simulink model "dvbs2hdlTransmitterCore"  (R2024b)
settings: Solver=FixedStepDiscrete  StartTime=0.0  StopTime=0  RelTol=1e-3
libraries: hdlsllib x105, simulink x41, dspsigops x7, commseqgen3 x5, whdlutilities x5, commhdlcrc x2, dsphdlfiltering2 x1, whdlmod x1
(part 1 of 5)
settings Model: DataDictionary=dvbs2hdlReceiverData.sldd  DataTypeOverride=Off  Creator=The MathWorks, Inc.  LastModifiedBy=daniel
settings SolverCC: MaxZcPerStep=1
settings OptimizationCC: BlockReduction=off  ConditionallyExecuteInputs=off  DefaultParameterBehavior=Inlined  InheritOutputTypeSmallerThanSingle=on  ReuseModelBlockBuffer=off
settings DebuggingCC: AlgebraicLoopMsg=error  SingleTaskRateTransMsg=error  SubsystemReferenceDiagnosticForUnitTest=warning
settings HardwareCC: ProdBitPerPointer=32  ProdBitPerSizeT=32  ProdBitPerPtrDiffT=32  ProdLargestAtomicFloat=None  ProdIntDivRoundTo=Undefined  ProdEndianess=Unspecified  ProdWordSize=32  ProdHWDeviceType=ASIC/FPGA->ASIC/FPGA  TargetBitPerLong=64  TargetBitPerPointer=64  TargetBitPerSizeT=64  TargetBitPerPtrDiffT=64  TargetLongLongMode=on  TargetIntDivRoundTo=Zero  TargetEndianess=LittleEndian  TargetWordSize=64  TargetHWDeviceType=Custom Processor->MATLAB Host Computer  ProdEqTarget=off
settings ModelReferenceCC: EnableRefExpFcnMdlSchedulingChecks=on
settings RTWCC: GPUComputeCapability=3.5  DLArmComputeVersion=19.05

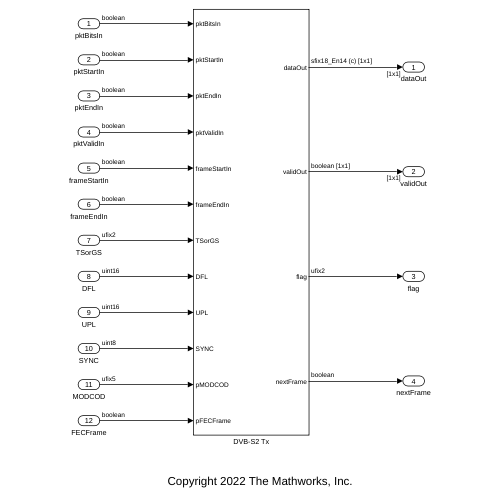
[thumbnail: Simulink's stored preview of the top-level diagram]
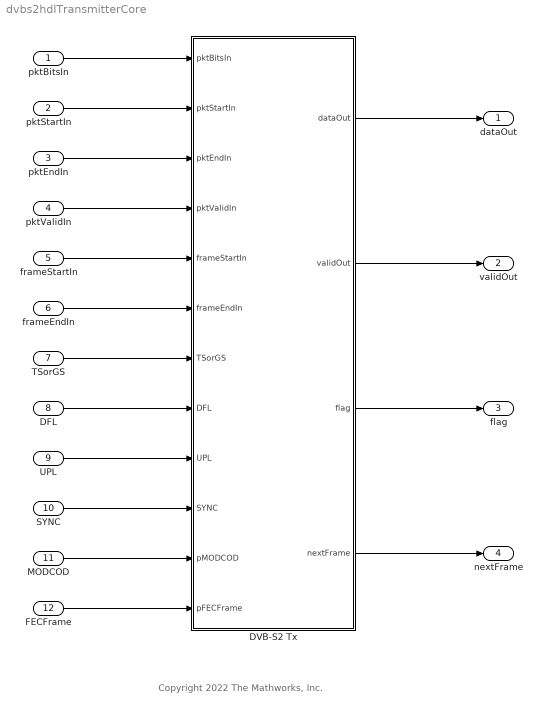
== system dvbs2hdlTransmitterCore ==
  note: Copyright 2022 The Mathworks, Inc.
  pktBitsIn : Inport  OutDataTypeStr=boolean  PortDimensions=1
  pktStartIn : Inport  Port=2  OutDataTypeStr=boolean  PortDimensions=1
  pktEndIn : Inport  Port=3  OutDataTypeStr=boolean  PortDimensions=1
  pktValidIn : Inport  Port=4  OutDataTypeStr=boolean  PortDimensions=1
  frameStartIn : Inport  Port=5  OutDataTypeStr=boolean  PortDimensions=1
  frameEndIn : Inport  Port=6  OutDataTypeStr=boolean  PortDimensions=1
  TSorGS : Inport  Port=7  OutDataTypeStr=fixdt(0,2,0)  PortDimensions=1
  DFL : Inport  Port=8  OutDataTypeStr=uint16  PortDimensions=1
  UPL : Inport  Port=9  OutDataTypeStr=uint16  PortDimensions=1
  SYNC : Inport  Port=10  OutDataTypeStr=uint8  PortDimensions=1
  MODCOD : Inport  Port=11  OutDataTypeStr=fixdt(0,5,0)  PortDimensions=1
  FECFrame : Inport  Port=12  OutDataTypeStr=boolean  PortDimensions=1
  DVB-S2 Tx : Subsystem  mask{Rsym=5e6}
      mask prompts: Rsym "Symbol Rate:"
      mask init:
      | config = dvbs2hdlTxParameters();
  dataOut : Outport
  validOut : Outport  Port=2
  flag : Outport  Port=3
  nextFrame : Outport  Port=4
  wires:
  pktBitsIn/1 -> DVB-S2 Tx/1(pktBitsIn)
  pktStartIn/1 -> DVB-S2 Tx/2(pktStartIn)
  pktEndIn/1 -> DVB-S2 Tx/3(pktEndIn)
  pktValidIn/1 -> DVB-S2 Tx/4(pktValidIn)
  frameStartIn/1 -> DVB-S2 Tx/5(frameStartIn)
  frameEndIn/1 -> DVB-S2 Tx/6(frameEndIn)
  TSorGS/1 -> DVB-S2 Tx/7(TSorGS)
  DFL/1 -> DVB-S2 Tx/8(DFL)
  UPL/1 -> DVB-S2 Tx/9(UPL)
  SYNC/1 -> DVB-S2 Tx/10(SYNC)
  MODCOD/1 -> DVB-S2 Tx/11(pMODCOD)
  FECFrame/1 -> DVB-S2 Tx/12(pFECFrame)
  DVB-S2 Tx/4(nextFrame) -> nextFrame/1
  DVB-S2 Tx/2(validOut) -> validOut/1
  DVB-S2 Tx/1(dataOut) -> dataOut/1
  DVB-S2 Tx/3(flag) -> flag/1

== system dvbs2hdlTransmitterCore/DVB-S2 Tx ==
  pktBitsIn : Inport  SampleTime=1/(Rsym*8)
  pktStartIn : Inport  Port=2
  pktEndIn : Inport  Port=3
  pktValidIn : Inport  Port=4
  frameStartIn : Inport  Port=5
  frameEndIn : Inport  Port=6
  TSorGS : Inport  Port=7
  DFL : Inport  Port=8
  UPL : Inport  Port=9
  SYNC : Inport  Port=10
  pMODCOD : Inport  Port=11
  pFECFrame : Inport  Port=12
  BB Frame Generator : Subsystem
  Bit Concat : hdlsllib/Logic and Bit Operations/Bit Concat  numInputs=2
  Delay : Delay  DelayLength=1
  FEC Encoder : Subsystem
  Interleaver : Subsystem
  Logical Operator : Logic  Operator=NOT  AllPortsSameDT=off  OutDataTypeStr=boolean
  Logical Operator1 : Logic  AllPortsSameDT=off  OutDataTypeStr=boolean
  MODCOD Source Coder : Subsystem
  No HDL : Subsystem
  PL Frame Generator : Subsystem
  RRC Transmit Filter : Subsystem
  Symbol Modulator : Subsystem
  Unit Delay Enabled Resettable Synchronous : hdlsllib/Discrete/Unit Delay Enabled Resettable Synchronous  InitialCondition=0.0  SampleTime=-1
  dataOut : Outport
  validOut : Outport  Port=2
  flag : Outport  Port=3
  nextFrame : Outport  Port=4
  wires:
  BB Frame Generator/4(validOut) -> MODCOD Source Coder/4(validIn)
  Delay/1 -> Logical Operator/1
  Logical Operator/1 -> Logical Operator1/2
  Logical Operator1/1 -> Unit Delay Enabled Resettable Synchronous/2, Unit Delay Enabled Resettable Synchronous/1
  PL Frame Generator/4(PLHeaderEnd) -> Bit Concat/2, No HDL/2(enb)
  PL Frame Generator/3(dummyHeaderEnd) -> Bit Concat/1, No HDL/1(Enable)
  Interleaver/8(MODCOD) -> Symbol Modulator/8(MODCOD)
  Interleaver/7(modIdx) -> Symbol Modulator/7(modIdx)
  Interleaver/6(codIdx) -> Symbol Modulator/6(codIdx)
  Interleaver/5(FECFrame) -> Symbol Modulator/5(FECFrame)
  Interleaver/4(validOut) -> Symbol Modulator/4(validIn)
  Interleaver/3(endOut) -> Symbol Modulator/3(endIn)
  Interleaver/2(startOut) -> Symbol Modulator/2(startIn)
  Interleaver/1(dataOut) -> Symbol Modulator/1(dataIn)
  FEC Encoder/7(MODCOD) -> Interleaver/7(MODCODIn)
  FEC Encoder/5(codOut) -> Interleaver/5(codIdxIn)
  FEC Encoder/2(validOut) -> Interleaver/2(validIn)
  FEC Encoder/1(dataOut) -> Interleaver/1(dataIn)
  PL Frame Generator/2(validOut) -> RRC Transmit Filter/2(validIn)
  PL Frame Generator/1(dataOut) -> RRC Transmit Filter/1(dataIn)
  Symbol Modulator/8(MODCODOut) -> PL Frame Generator/8(modcod)
  Symbol Modulator/7(FECFrameOut) -> PL Frame Generator/7(fecframeIn)
  Symbol Modulator/6(codIdxOut) -> PL Frame Generator/6(codIdxIn)
  Symbol Modulator/5(modIdxOut) -> PL Frame Generator/5(modIdxIn)
  Symbol Modulator/4(validOut) -> PL Frame Generator/4(validIn)
  Symbol Modulator/3(endOut) -> PL Frame Generator/3(endIn)
  Symbol Modulator/2(startOut) -> PL Frame Generator/2(startIn)
  Symbol Modulator/1(dataOut) -> PL Frame Generator/1(dataIn)
  RRC Transmit Filter/2(validOut) -> validOut/1
  RRC Transmit Filter/1(dataOut) -> dataOut/1
  pFECFrame/1 -> BB Frame Generator/12(pFECFrame)
  Interleaver/9(ready) -> Delay/1, Logical Operator1/1
  frameEndIn/1 -> BB Frame Generator/6(frameEndIn)
  TSorGS/1 -> BB Frame Generator/7(TSorGS)
  pktBitsIn/1 -> BB Frame Generator/1(pktBitsIn)
  pktEndIn/1 -> BB Frame Generator/3(pktEndIn)
  DFL/1 -> BB Frame Generator/8(DFL)
  FEC Encoder/3(startOut) -> Interleaver/3(paramValid)
  MODCOD Source Coder/4(validOut) -> FEC Encoder/4(validIn)
  pktValidIn/1 -> BB Frame Generator/4(pktValidIn)
  MODCOD Source Coder/1(dataOut) -> FEC Encoder/1(dataIn)
  MODCOD Source Coder/3(endOut) -> FEC Encoder/3(endIn)
  MODCOD Source Coder/8(MODCOD) -> FEC Encoder/8(MODCODIn)
  BB Frame Generator/6(FECFrame) -> MODCOD Source Coder/6(FECFrameIn)
  BB Frame Generator/1(dataOut) -> MODCOD Source Coder/1(dataIn)
  pMODCOD/1 -> BB Frame Generator/11(pMODCOD)
  MODCOD Source Coder/2(startOut) -> FEC Encoder/2(startIn)
  MODCOD Source Coder/6(codeRateIdx) -> FEC Encoder/6(codeRateIdxIn)
  SYNC/1 -> BB Frame Generator/10(SYNC)
  UPL/1 -> BB Frame Generator/9(UPL)
  BB Frame Generator/2(startOut) -> MODCOD Source Coder/2(startIn)
  pktStartIn/1 -> BB Frame Generator/2(pktStartIn)
  BB Frame Generator/5(MODCOD) -> MODCOD Source Coder/5(MODCODIn)
  MODCOD Source Coder/5(modIdx) -> FEC Encoder/5(modIdxIn)
  MODCOD Source Coder/7(FECFrame) -> FEC Encoder/7(FECFrameIn)
  frameStartIn/1 -> Unit Delay Enabled Resettable Synchronous/3, BB Frame Generator/5(frameStartIn)
  FEC Encoder/4(modOut) -> Interleaver/4(modIdxIn)
  BB Frame Generator/3(endOut) -> MODCOD Source Coder/3(endIn)
  FEC Encoder/6(fecOut) -> Interleaver/6(fecframeIn)
  Unit Delay Enabled Resettable Synchronous/1 -> nextFrame/1
  Bit Concat/1 -> flag/1

== system dvbs2hdlTransmitterCore/DVB-S2 Tx/BB Frame Generator ==
  pktBitsIn : Inport
  pktStartIn : Inport  Port=2
  pktEndIn : Inport  Port=3
  pktValidIn : Inport  Port=4
  frameStartIn : Inport  Port=5
  frameEndIn : Inport  Port=6
  TSorGS : Inport  Port=7
  DFL : Inport  Port=8
  UPL : Inport  Port=9
  SYNC : Inport  Port=10
  pMODCOD : Inport  Port=11
  pFECFrame : Inport  Port=12
  BB Header and Data CRC Generator : Subsystem
  BB Scrambler : Subsystem
  Data Store FIFO : Subsystem
  Delay{,1..5} (6 alike) : Delay  DelayLength=1
  Multiplexer : Subsystem
  Unit Delay Enabled Synchronous{,1..5} (6 alike) : hdlsllib/Discrete/Unit Delay Enabled Synchronous  InitialCondition=0.0  SampleTime=-1
  dataOut : Outport
  startOut : Outport  Port=2
  endOut : Outport  Port=3
  validOut : Outport  Port=4
  MODCOD : Outport  Port=5
  FECFrame : Outport  Port=6
  wires:
  BB Scrambler/6(FECFrameOut) -> FECFrame/1
  Multiplexer/6(FECFrameOut) -> BB Scrambler/6(FECFrame)
  Data Store FIFO/8(FECFrameOut) -> Multiplexer/8(FECFrame)
  BB Header and Data CRC Generator/9(FECFrameOut) -> Data Store FIFO/9(FECFrame)
  Unit Delay Enabled Synchronous5/1 -> BB Header and Data CRC Generator/12(FECFrame)
  pFECFrame/1 -> Unit Delay Enabled Synchronous5/1
  BB Scrambler/5(MODCODOut) -> MODCOD/1
  Multiplexer/5(MODCODOut) -> BB Scrambler/5(MODCOD)
  Data Store FIFO/7(MODCODOut) -> Multiplexer/7(MODCOD)
  BB Header and Data CRC Generator/8(MODCODOut) -> Data Store FIFO/8(MODCOD)
  pMODCOD/1 -> Unit Delay Enabled Synchronous4/1
  Unit Delay Enabled Synchronous4/1 -> BB Header and Data CRC Generator/11(MODCOD)
  BB Header and Data CRC Generator/7(validOut) -> Data Store FIFO/7(validOut)
  BB Header and Data CRC Generator/6(endOut) -> Data Store FIFO/6(endOut)
  BB Header and Data CRC Generator/5(startOut) -> Data Store FIFO/5(startOut)
  BB Header and Data CRC Generator/4(bitsOut) -> Data Store FIFO/4(bitsOut)
  Data Store FIFO/6(headerValid) -> Multiplexer/6(headerValid)
  Data Store FIFO/5(headerStart) -> Multiplexer/5(headerStart)
  Data Store FIFO/4(headerBits) -> Multiplexer/4(headerBits)
  Data Store FIFO/3(dataEnd) -> Multiplexer/3(dataEnd)
  Data Store FIFO/2(dataValid) -> Multiplexer/2(dataValid)
  Data Store FIFO/1(dataBits) -> Multiplexer/1(dataBits)
  BB Header and Data CRC Generator/3(DFLOut) -> Data Store FIFO/3(DFLOut)
  BB Header and Data CRC Generator/2(pktValid) -> Data Store FIFO/2(pktValid)
  BB Header and Data CRC Generator/1(pktBits) -> Data Store FIFO/1(pktBits)
  Unit Delay Enabled Synchronous3/1 -> BB Header and Data CRC Generator/10(SYNC)
  Unit Delay Enabled Synchronous2/1 -> BB Header and Data CRC Generator/9(UPL)
  Unit Delay Enabled Synchronous/1 -> BB Header and Data CRC Generator/8(DFL)
  Unit Delay Enabled Synchronous1/1 -> BB Header and Data CRC Generator/7(TSorGS)
  Delay2/1 -> BB Header and Data CRC Generator/6(frameStart)
  Delay/1 -> BB Header and Data CRC Generator/5(frameEnd)
  Delay1/1 -> BB Header and Data CRC Generator/4(validIn)
  Delay3/1 -> BB Header and Data CRC Generator/3(endIn)
  Delay4/1 -> BB Header and Data CRC Generator/2(startIn)
  Delay5/1 -> BB Header and Data CRC Generator/1(dataIn)
  BB Scrambler/4(validOut) -> validOut/1
  BB Scrambler/3(endOut) -> endOut/1
  BB Scrambler/2(startOut) -> startOut/1
  BB Scrambler/1(bitsOut) -> dataOut/1
  Multiplexer/1(dataOut) -> BB Scrambler/1(bitsIn)
  Multiplexer/3(endOut) -> BB Scrambler/3(endIn)
  Multiplexer/2(startOut) -> BB Scrambler/2(startIn)
  Multiplexer/4(validOut) -> BB Scrambler/4(validIn)
  frameStartIn/1 -> Delay2/1, Unit Delay Enabled Synchronous1/2, Unit Delay Enabled Synchronous/2, Unit Delay Enabled Synchronous2/2, Unit Delay Enabled Synchronous3/2, Unit Delay Enabled Synchronous4/2, Unit Delay Enabled Synchronous5/2
  pktBitsIn/1 -> Delay5/1
  pktStartIn/1 -> Delay4/1
  pktEndIn/1 -> Delay3/1
  pktValidIn/1 -> Delay1/1
  frameEndIn/1 -> Delay/1
  DFL/1 -> Unit Delay Enabled Synchronous/1
  UPL/1 -> Unit Delay Enabled Synchronous2/1
  SYNC/1 -> Unit Delay Enabled Synchronous3/1
  TSorGS/1 -> Unit Delay Enabled Synchronous1/1

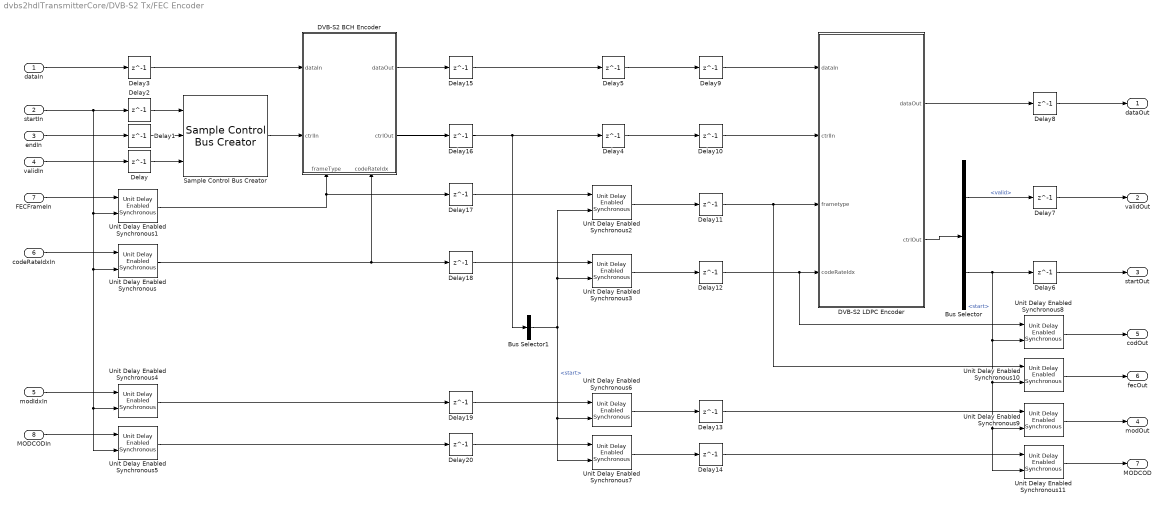
== system dvbs2hdlTransmitterCore/DVB-S2 Tx/FEC Encoder ==
  dataIn : Inport
  startIn : Inport  Port=2
  endIn : Inport  Port=3
  validIn : Inport  Port=4
  modIdxIn : Inport  Port=5
  codeRateIdxIn : Inport  Port=6
  FECFrameIn : Inport  Port=7
  MODCODIn : Inport  Port=8
  Bus Selector : BusSelector  OutputSignals=valid,start
  Bus Selector1 : BusSelector  OutputSignals=start
  DVB-S2 BCH Encoder : Subsystem
      settings: PortSchema="{\"entries\":[{\"content\":{\"sides\":[{\"content\":{\"connectorIds\":[\"In1\",\"In2\"]},\"type\":\"ConnectorPlacement.EquallySpacedRectSide\",\"uuid\":\"13af3286-4637-4d72-a307-8c85e9ac2c6a\"},{\"content\":{\"connectorIds\":[\"Out1\",\"Out2\"],\"side\":\"RIGHT\"},\"type\":\"ConnectorPlacement.EquallySpacedRectSide\",\"uuid\":\"54f73aa5-b2da-4ba3-a1a2-5182494cfccf\"},{\"content\":{\"connectorIds\":[],\"side\":\"TOP\"},\"type\":\"ConnectorPlacement.EquallySpacedRectSide\",\"uuid\":\"2ea82380-bfbe-4164-83be-b799e77a8d24\"},{\"content\":{\"connectorIds\":[\"In3\",\"In4\"],\"side\":\"BOTTOM\"},\"type\":\"ConnectorPlacement.EquallySpacedRectSide\",\"uuid\":\"b02c2a1c-1695-4c1d-92ad-7323b1632720\"}]},\"type\":\"ConnectorPlacement.EquallySpacedConnector\",\"uuid\":\"56402870-0df7-4074-88cd-682c42d8a6b3\"}],\"packageUris\":[\"http://schema.mathworks.com/mf0/Connector/R2020b\"],\"version\":\"1.0\"}"
  DVB-S2 LDPC Encoder : Subsystem
      mask init:
      | config = dvbs2hdlTxParameters();
      | columnSum = config.LDPCcolumnSum;  %#ok<NASGU> 
      | ramLUT    = config.LDPCramLUT;     %#ok<NASGU> 
      | shiftLUT  = config.LDPCshiftLUT;   %#ok<NASGU>
  Delay{,1..20} (21 alike) : Delay  DelayLength=1
  Sample Control Bus Creator : whdlutilities/Sample Control Bus Creator
  Unit Delay Enabled Synchronous{,1..11} (12 alike) : hdlsllib/Discrete/Unit Delay Enabled Synchronous  InitialCondition=0.0  SampleTime=-1
  dataOut : Outport
  validOut : Outport  Port=2
  startOut : Outport  Port=3
  modOut : Outport  Port=4
  codOut : Outport  Port=5
  fecOut : Outport  Port=6
  MODCOD : Outport  Port=7
  wires:
  Delay20/1 -> Unit Delay Enabled Synchronous7/1
  Delay19/1 -> Unit Delay Enabled Synchronous6/1
  Delay18/1 -> Unit Delay Enabled Synchronous3/1
  Delay17/1 -> Unit Delay Enabled Synchronous2/1
  Delay16/1 -> Delay4/1, Bus Selector1/1
  Delay15/1 -> Delay5/1
  Delay14/1 -> Unit Delay Enabled Synchronous11/1
  Delay13/1 -> Unit Delay Enabled Synchronous9/1
  Delay12/1 -> DVB-S2 LDPC Encoder/4(codeRateIdx), Unit Delay Enabled Synchronous8/1
  Delay11/1 -> DVB-S2 LDPC Encoder/3(frametype), Unit Delay Enabled Synchronous10/1
  Delay10/1 -> DVB-S2 LDPC Encoder/2(ctrlIn)
  Delay9/1 -> DVB-S2 LDPC Encoder/1(dataIn)
  validIn/1 -> Delay/1
  endIn/1 -> Delay1/1
  startIn/1 -> Delay2/1, Unit Delay Enabled Synchronous1/2, Unit Delay Enabled Synchronous/2, Unit Delay Enabled Synchronous4/2, Unit Delay Enabled Synchronous5/2
  Delay3/1 -> DVB-S2 BCH Encoder/1(dataIn)
  Unit Delay Enabled Synchronous1/1 -> Delay17/1, DVB-S2 BCH Encoder/3(frameType)
  Unit Delay Enabled Synchronous/1 -> DVB-S2 BCH Encoder/4(codeRateIdx), Delay18/1
  Sample Control Bus Creator/1 -> DVB-S2 BCH Encoder/2(ctrlIn)
  DVB-S2 BCH Encoder/2(ctrlOut) -> Delay16/1
  DVB-S2 BCH Encoder/1(dataOut) -> Delay15/1
  Unit Delay Enabled Synchronous3/1 -> Delay12/1
  Delay8/1 -> dataOut/1
  Delay7/1 -> validOut/1
  Delay6/1 -> startOut/1
  Delay5/1 -> Delay9/1
  Delay4/1 -> Delay10/1
  Delay2/1 -> Sample Control Bus Creator/1
  Delay1/1 -> Sample Control Bus Creator/2
  Delay/1 -> Sample Control Bus Creator/3
  Unit Delay Enabled Synchronous7/1 -> Delay14/1
  Unit Delay Enabled Synchronous6/1 -> Delay13/1
  Unit Delay Enabled Synchronous11/1 -> MODCOD/1
  Unit Delay Enabled Synchronous10/1 -> fecOut/1
  Unit Delay Enabled Synchronous9/1 -> modOut/1
  Unit Delay Enabled Synchronous8/1 -> codOut/1
  Unit Delay Enabled Synchronous5/1 -> Delay20/1
  Unit Delay Enabled Synchronous4/1 -> Delay19/1
  MODCODIn/1 -> Unit Delay Enabled Synchronous5/1
  Unit Delay Enabled Synchronous2/1 -> Delay11/1
  Bus Selector1/1 -> Unit Delay Enabled Synchronous6/2, Unit Delay Enabled Synchronous7/2, Unit Delay Enabled Synchronous3/2, Unit Delay Enabled Synchronous2/2  "<start>"
  dataIn/1 -> Delay3/1
  codeRateIdxIn/1 -> Unit Delay Enabled Synchronous/1
  FECFrameIn/1 -> Unit Delay Enabled Synchronous1/1
  modIdxIn/1 -> Unit Delay Enabled Synchronous4/1
  Bus Selector/2 -> Delay6/1, Unit Delay Enabled Synchronous8/2, Unit Delay Enabled Synchronous10/2, Unit Delay Enabled Synchronous9/2, Unit Delay Enabled Synchronous11/2  "<start>"
  Bus Selector/1 -> Delay7/1  "<valid>"
  DVB-S2 LDPC Encoder/2(ctrlOut) -> Bus Selector/1
  DVB-S2 LDPC Encoder/1(dataOut) -> Delay8/1

== system dvbs2hdlTransmitterCore/DVB-S2 Tx/Interleaver ==
  dataIn : Inport
  validIn : Inport  Port=2
  paramValid : Inport  Port=3
  modIdxIn : Inport  Port=4
  codIdxIn : Inport  Port=5
  fecframeIn : Inport  Port=6
  MODCODIn : Inport  Port=7
  DVB-S2 HDL Interleaver : Subsystem  mask{mode=Interleaver 8x, Tsamp=1/(Rsym*8)}
      mask prompts: mode "Mode :"; Tsamp "Sample Time"
      mask init:
      | switch mode
      |     case 1
      |         isInterleave = true;
      |     case 2
      |         isInterleave = false;
      |     otherwise
      |         error(['Invalid mode of ' mode]);
      | end
      | clear mode;
      | 
      | ConfigRx.RAMCapacity = 64800*2;
      | ConfigRx.ShortFrameLen = 16200;
      | ConfigRx.NormalFrameLen = 64800;
      mask TypeOptions mode: Interleaver 8x | Deinterleaver
      mask Display: disp(['DVB-S2' newline 'HDL ' newline get_param(gcb,'mode')]);
  Delay{1,3..5,17..20} (8 alike) : Delay  DelayLength=8
  Delay{2,6..13} (9 alike) : Delay  DelayLength=1
  Unit Delay Enabled Synchronous : hdlsllib/Discrete/Unit Delay Enabled Synchronous  InitialCondition=0.0  SampleTime=-1
  dataOut : Outport
  startOut : Outport  Port=2
  endOut : Outport  Port=3
  validOut : Outport  Port=4
  FECFrame : Outport  Port=5
  codIdx : Outport  Port=6
  modIdx : Outport  Port=7
  MODCOD : Outport  Port=8
  ready : Outport  Port=9
  wires:
  Delay1/1 -> endOut/1
  fecframeIn/1 -> DVB-S2 HDL Interleaver/6(fecframeIn)
  modIdxIn/1 -> DVB-S2 HDL Interleaver/4(modIdxIn)
  codIdxIn/1 -> DVB-S2 HDL Interleaver/5(codIdxIn)
  Delay4/1 -> validOut/1
  DVB-S2 HDL Interleaver/8(ready) -> ready/1
  MODCODIn/1 -> Unit Delay Enabled Synchronous/1
  Delay17/1 -> FECFrame/1
  Delay5/1 -> startOut/1
  Delay10/1 -> DVB-S2 HDL Interleaver/2(validIn)
  Delay19/1 -> dataOut/1
  Delay12/1 -> Delay18/1
  dataIn/1 -> Delay9/1
  Delay20/1 -> modIdx/1
  DVB-S2 HDL Interleaver/1(rd_dout) -> Delay2/1
  Delay11/1 -> Delay17/1
  validIn/1 -> Delay10/1
  Delay9/1 -> DVB-S2 HDL Interleaver/1(dataIn)
  Delay8/1 -> Delay4/1
  Delay2/1 -> Delay19/1
  Unit Delay Enabled Synchronous/1 -> Delay3/1
  DVB-S2 HDL Interleaver/2(rd_startOut) -> Delay6/1, Unit Delay Enabled Synchronous/2
  DVB-S2 HDL Interleaver/6(codIdx) -> Delay12/1
  DVB-S2 HDL Interleaver/3(rd_endOut) -> Delay7/1
  Delay3/1 -> MODCOD/1
  Delay6/1 -> Delay5/1
  Delay18/1 -> codIdx/1
  DVB-S2 HDL Interleaver/7(modIdx) -> Delay13/1
  Delay7/1 -> Delay1/1
  paramValid/1 -> DVB-S2 HDL Interleaver/3(paramValid)
  DVB-S2 HDL Interleaver/4(rd_validOut) -> Delay8/1
  DVB-S2 HDL Interleaver/5(fecframe) -> Delay11/1
  Delay13/1 -> Delay20/1

== system dvbs2hdlTransmitterCore/DVB-S2 Tx/MODCOD Source Coder ==
  dataIn : Inport
  startIn : Inport  Port=2
  endIn : Inport  Port=3
  validIn : Inport  Port=4
  MODCODIn : Inport  Port=5
  FECFrameIn : Inport  Port=6
  Data Type Conversion : DataTypeConversion  OutDataTypeStr=fixdt(0,4,0)  SaturateOnIntegerOverflow=off  RndMeth=Floor
  Data Type Conversion1 : DataTypeConversion  OutDataTypeStr=boolean  SaturateOnIntegerOverflow=off  RndMeth=Floor
  Data Type Conversion2 : DataTypeConversion  OutDataTypeStr=fixdt(0,2,0)  SaturateOnIntegerOverflow=off  RndMeth=Floor
  Data Type Conversion3 : DataTypeConversion  OutDataTypeStr=fixdt(0,5,0)  SaturateOnIntegerOverflow=off  RndMeth=Floor
  Delay{7..8,14..16} (5 alike) : Delay  DelayLength=1
  Unit Delay Enabled Synchronous : hdlsllib/Discrete/Unit Delay Enabled Synchronous  InitialCondition=0.0  SampleTime=-1
  convertMODCOD : MATLAB Function  TreatAsAtomicUnit=on
  dataOut : Outport
  startOut : Outport  Port=2
  endOut : Outport  Port=3
  validOut : Outport  Port=4
  modIdx : Outport  Port=5
  codeRateIdx : Outport  Port=6
  FECFrame : Outport  Port=7
  MODCOD : Outport  Port=8
  wires:
  Data Type Conversion2/1 -> modIdx/1
  Data Type Conversion1/1 -> FECFrame/1
  Data Type Conversion/1 -> codeRateIdx/1
  Delay7/1 -> dataOut/1
  Delay8/1 -> startOut/1
  endIn/1 -> Delay14/1
  Data Type Conversion3/1 -> MODCOD/1
  validIn/1 -> Delay15/1
  dataIn/1 -> Delay7/1
  Delay14/1 -> endOut/1
  FECFrameIn/1 -> Delay16/1
  convertMODCOD/1(modIdx) -> Data Type Conversion2/1
  MODCODIn/1 -> Unit Delay Enabled Synchronous/1
  Delay15/1 -> validOut/1
  Unit Delay Enabled Synchronous/1 -> convertMODCOD/1(modcod), Data Type Conversion3/1
  convertMODCOD/2(codIdx) -> Data Type Conversion/1
  startIn/1 -> Delay8/1, Unit Delay Enabled Synchronous/2
  Delay16/1 -> Data Type Conversion1/1

== system dvbs2hdlTransmitterCore/DVB-S2 Tx/No HDL ==
  Enable : Inport
  enb : Inport  Port=2
  HDL Counter : hdlsllib/Sources/HDL Counter  CountType=Free running  CountInit=0  CountStep=1  CountMax=25  CountFromType=Initial value  CountFrom=0  CountResetPort=off  CountLoadPort=off  CountEnbPort=on  CountDirPort=off  CountHitOutputPort=off  CountDataType=Unsigned  CountWordLen=32  CountFracLen=0  CountSampTime=1
  Subsystem : Subsystem
  wires:
  Enable/1 -> Subsystem/Enable
  enb/1 -> HDL Counter/1
  HDL Counter/1 -> Subsystem/1(In1)

== system dvbs2hdlTransmitterCore/DVB-S2 Tx/PL Frame Generator ==
  dataIn : Inport
  startIn : Inport  Port=2
  endIn : Inport  Port=3
  validIn : Inport  Port=4
  modIdxIn : Inport  Port=5
  codIdxIn : Inport  Port=6
  fecframeIn : Inport  Port=7
  modcod : Inport  Port=8
  16x : MATLAB Function  TreatAsAtomicUnit=on
  Constant2 : Constant  Value=true  SampleTime=2/(Rsym)
  Delay : Delay  DelayLength=1
  Delay{1,3,7..11} (7 alike) : Delay  DelayLength=37
  Delay2 : Delay  DelayLength=1
  Downsample : DownSample  N=16  RateOptions=Allow multirate processing
  Downsample{1..2,5..6} (4 alike) : DownSample  N=8  RateOptions=Allow multirate processing
  Downsample3 : DownSample  N=16  RateOptions=Allow multirate processing
  Downsample4 : DownSample  N=16  RateOptions=Allow multirate processing
  Frame Length : Subsystem
  Multiplexer : Subsystem
  PL Data Scrambler : Subsystem
  PL Header Generator : Subsystem
  RAM FIFO : Subsystem
  Subsystem : Subsystem
  Terminator : Terminator
  dataOut : Outport
  validOut : Outport  Port=2
  dummyHeaderEnd : Outport  Port=3
  PLHeaderEnd : Outport  Port=4
  wires:
  16x/1(validOut) -> Downsample/1
  Constant2/1 -> PL Header Generator/2(pilotActive)
  Downsample/1 -> PL Header Generator/1(trigger)
  modcod/1 -> Downsample4/1
  startIn/1 -> Delay1/1, 16x/1(trigger)
  Delay2/1 -> RAM FIFO/2(validIn)
  modIdxIn/1 -> Delay9/1
  PL Header Generator/2(validOut) -> Delay2/1
  PL Header Generator/1(dataOut) -> Delay/1
  codIdxIn/1 -> Delay10/1
  fecframeIn/1 -> Delay11/1, Downsample3/1
  validIn/1 -> Delay8/1
  dataIn/1 -> Delay7/1
  Downsample3/1 -> PL Header Generator/4(fecframe)
  Downsample4/1 -> PL Header Generator/3(modcod)
  Frame Length/1(xFECFrameLength) -> Downsample5/1
  RAM FIFO/10(slotsValid) -> Multiplexer/10(slotsValid)
  RAM FIFO/7(pilotValid) -> Multiplexer/7(pilotValid)
  RAM FIFO/4(plheaderValid) -> Multiplexer/4(plheaderValid)
  Delay/1 -> RAM FIFO/1(dataIn)
  Downsample1/1 -> RAM FIFO/3(dataIn1)
  Downsample2/1 -> RAM FIFO/5(validIn1)
  Downsample5/1 -> RAM FIFO/6(frameLength)
  Downsample6/1 -> RAM FIFO/4(startIn1)
  RAM FIFO/1(plheaderData) -> Multiplexer/1(plheaderData)
  RAM FIFO/2(plheaderStart) -> Multiplexer/2(plheaderStart)
  RAM FIFO/5(pilotData) -> Multiplexer/5(pilotdata)
  RAM FIFO/6(pilotEnd) -> Multiplexer/6(pilotEnd)
  RAM FIFO/8(slotsData) -> Multiplexer/8(slotsData)
  RAM FIFO/9(data16SlotsEnd) -> Multiplexer/9(data16SlotsEnd)
  RAM FIFO/3(plheaderEnd) -> Multiplexer/3(plheaderEnd), PLHeaderEnd/1
  Delay11/1 -> Frame Length/1(fecframe)
  Delay9/1 -> Frame Length/2(modIdx)
  Delay10/1 -> Terminator/1
  Delay7/1 -> Subsystem/1(data)
  Delay1/1 -> Subsystem/2(start)
  Delay8/1 -> Subsystem/4(validIn)
  Subsystem/1(dataOut) -> Downsample1/1
  Subsystem/2(startOut) -> Downsample6/1
  Subsystem/3(validOut) -> Downsample2/1
  endIn/1 -> Delay3/1
  Delay3/1 -> Subsystem/3(endIn)
  RAM FIFO/11(dummyData) -> Multiplexer/11(dummyData)
  RAM FIFO/12(dummyValid) -> Multiplexer/12(dummyValid)
  RAM FIFO/13(dummyHeaderSrt) -> Multiplexer/13(dummyHeaderSrt)
  RAM FIFO/14(dummyHeaderEnd) -> Multiplexer/14(dummyHeaderEnd), dummyHeaderEnd/1
  PL Data Scrambler/2(validOut) -> validOut/1
  Multiplexer/3(endOfPlheader) -> PL Data Scrambler/3(endOfPlheader)
  Multiplexer/2(startOfPlheader) -> PL Data Scrambler/2(startOfPlheader)
  Multiplexer/4(validOut) -> PL Data Scrambler/4(validIn)
  PL Data Scrambler/1(dataOut) -> dataOut/1
  Multiplexer/1(dataOut) -> PL Data Scrambler/1(dataIn)

== system dvbs2hdlTransmitterCore/DVB-S2 Tx/RRC Transmit Filter ==
  dataIn : Inport
  validIn : Inport  Port=2
  Discrete FIR Filter : dsphdlfiltering2/Discrete FIR Filter  NumeratorSource=Property  Numerator=config.RRCImpulseResponse  NumeratorPrototype=[]  FilterStructure=Direct form systolic  SerializationOption=Minimum number of cycles between valid input samples  NumCycles=2  NumberOfMultipliers=2  SimulateUsing=Code generation  roundingMode=Floor  overflowMode=off  CoefficientsDataTypeStr=Inherit: Same word length as input  OutputDataTypeStr=Inherit: Same word length as input  ResetInputPort=off  HDLGlobalReset=off  CoeffMultiplier=Multiplier  UseMultForPow2Coeff=on
  Repeat : dspsigops/Repeat  FactorSource=Dialog parameter  N=config.SamplesPerSymbol  Nmax=16  RateOptions=Allow multirate processing  ic=0  mode=Unused parameter value
      settings: LibrarySourceBlock=dsphdlsupportsigops/Repeat
  Upsample : dspsigops/Upsample  FactorSource=Dialog parameter  N=config.SamplesPerSymbol  Nmax=16  phase=0  RateOptions=Allow multirate processing  ic=0  mode=Unused parameter value
      settings: LibrarySourceBlock=dsphdlsupportsigops/Upsample
  dataOut : Outport
  validOut : Outport  Port=2
  wires:
  Discrete FIR Filter/2 -> validOut/1
  Discrete FIR Filter/1 -> dataOut/1
  dataIn/1 -> Upsample/1
  Upsample/1 -> Discrete FIR Filter/1
  validIn/1 -> Repeat/1
  Repeat/1 -> Discrete FIR Filter/2

== system dvbs2hdlTransmitterCore/DVB-S2 Tx/Symbol Modulator ==
  dataIn : Inport
  startIn : Inport  Port=2
  endIn : Inport  Port=3
  validIn : Inport  Port=4
  FECFrame : Inport  Port=5
  codIdx : Inport  Port=6
  modIdx : Inport  Port=7
  MODCOD : Inport  Port=8
  DVB-S2 Symbol Modulator1 : whdlmod/DVB-S2 Symbol Modulator  ModulationSourceParams=Input port  ModulationScheme=QPSK  CodeRateAPSK=3/4  UnitAveragePower=off  SimulateUsing=Code generation  OutputDataType=Custom  WordLength=16
  Data Type Conversion : DataTypeConversion  OutDataTypeStr=fixdt(0,3,0)  SaturateOnIntegerOverflow=off  RndMeth=Floor
  Delay{,1..6,11,13} (9 alike) : Delay  DelayLength=1
  Delay{7..10,12,14} (6 alike) : Delay  DelayLength=3
  Delay{15..22} (8 alike) : Delay
  dataOut : Outport
  startOut : Outport  Port=2
  endOut : Outport  Port=3
  validOut : Outport  Port=4
  modIdxOut : Outport  Port=5
  codIdxOut : Outport  Port=6
  FECFrameOut : Outport  Port=7
  MODCODOut : Outport  Port=8
  wires:
  Data Type Conversion/1 -> DVB-S2 Symbol Modulator1/3
  DVB-S2 Symbol Modulator1/2 -> Delay16/1
  DVB-S2 Symbol Modulator1/1 -> Delay15/1
  Delay6/1 -> DVB-S2 Symbol Modulator1/5
  Delay1/1 -> DVB-S2 Symbol Modulator1/2
  Delay2/1 -> DVB-S2 Symbol Modulator1/1
  Delay22/1 -> FECFrameOut/1
  Delay21/1 -> MODCODOut/1
  Delay20/1 -> codIdxOut/1
  Delay19/1 -> modIdxOut/1
  Delay18/1 -> endOut/1
  Delay17/1 -> startOut/1
  Delay16/1 -> validOut/1
  Delay15/1 -> dataOut/1
  Delay14/1 -> Delay18/1
  Delay13/1 -> Delay14/1
  Delay12/1 -> Delay17/1
  Delay11/1 -> Delay12/1
  Delay10/1 -> Delay22/1
  Delay9/1 -> Delay21/1
  Delay8/1 -> Delay20/1
  Delay7/1 -> Delay19/1
  endIn/1 -> Delay13/1
  Delay5/1 -> Delay10/1
  FECFrame/1 -> Delay5/1
  Delay4/1 -> Delay9/1
  MODCOD/1 -> Delay4/1
  Delay3/1 -> Delay8/1, DVB-S2 Symbol Modulator1/4
  codIdx/1 -> Delay3/1
  startIn/1 -> Delay6/1, Delay11/1
  dataIn/1 -> Delay2/1
  validIn/1 -> Delay1/1
  Delay/1 -> Delay7/1, Data Type Conversion/1
  modIdx/1 -> Delay/1

== system dvbs2hdlTransmitterCore/DVB-S2 Tx/BB Frame Generator/BB Header and Data CRC Generator ==
  dataIn : Inport
  startIn : Inport  Port=2
  endIn : Inport  Port=3
  validIn : Inport  Port=4
  frameEnd : Inport  Port=5
  frameStart : Inport  Port=6
  TSorGS : Inport  Port=7
  DFL : Inport  Port=8
  UPL : Inport  Port=9
  SYNC : Inport  Port=10
  MODCOD : Inport  Port=11
  FECFrame : Inport  Port=12
  BB Header Generator : Subsystem
  Data Field Generator : Subsystem
  Delay{,1..10} (11 alike) : Delay  DelayLength=1
  Logical Operator : Logic  Operator=OR  AllPortsSameDT=off  OutDataTypeStr=boolean
  Logical Operator1 : Logic  AllPortsSameDT=off  OutDataTypeStr=boolean
  Logical Operator2 : Logic  Operator=NOT  AllPortsSameDT=off  OutDataTypeStr=boolean
  MATLAB Function : MATLAB Function  TreatAsAtomicUnit=on
  No HDL : Subsystem
      settings: PortSchema="{\"entries\":[{\"content\":{\"sides\":[{\"content\":{\"connectorIds\":[\"In1\",\"In2\"]},\"type\":\"ConnectorPlacement.EquallySpacedRectSide\",\"uuid\":\"2b0d8642-5d0a-4928-807b-7bdaa72465a7\"},{\"content\":{\"connectorIds\":[\"In3\"],\"side\":\"RIGHT\"},\"type\":\"ConnectorPlacement.EquallySpacedRectSide\",\"uuid\":\"c3d25bc5-ada1-46aa-97a0-2934df92f89e\"},{\"content\":{\"side\":\"TOP\"},\"type\":\"ConnectorPlacement.EquallySpacedRectSide\",\"uuid\":\"4e9ad39f-657b-49f8-9193-07411e04c0d0\"},{\"content\":{\"side\":\"BOTTOM\"},\"type\":\"ConnectorPlacement.EquallySpacedRectSide\",\"uuid\":\"c9ac8116-ea00-4596-919b-501b9f95d4cb\"}]},\"type\":\"ConnectorPlacement.EquallySpacedConnector\",\"uuid\":\"3e308e49-dc99-4f24-8c75-1c979d051dde\"}],\"packageUris\":[\"http://schema.mathworks.com/mf0/Connector/R2020b\"],\"version\":\"1.0\"}"
  pktBits : Outport
  pktValid : Outport  Port=2
  DFLOut : Outport  Port=3
  bitsOut : Outport  Port=4
  startOut : Outport  Port=5
  endOut : Outport  Port=6
  validOut : Outport  Port=7
  MODCODOut : Outport  Port=8
  FECFrameOut : Outport  Port=9
  wires:
  Delay10/1 -> FECFrameOut/1
  BB Header Generator/7(FECFrameOut) -> Delay10/1
  FECFrame/1 -> BB Header Generator/7(FECFrame)
  Delay9/1 -> MODCODOut/1
  Delay8/1 -> endOut/1
  Delay7/1 -> validOut/1
  Delay6/1 -> startOut/1
  Delay5/1 -> bitsOut/1
  Delay4/1 -> MATLAB Function/4(DFL), DFLOut/1
  Delay3/1 -> MATLAB Function/3(endIn)
  Delay2/1 -> MATLAB Function/2(startIn)
  Delay1/1 -> Logical Operator/1, MATLAB Function/1(validIn)
  Delay/1 -> Logical Operator1/1
  MODCOD/1 -> BB Header Generator/6(MODCOD)
  BB Header Generator/6(MODCODOut) -> Delay9/1
  Logical Operator/1 -> pktValid/1
  Logical Operator1/1 -> pktBits/1
  Logical Operator2/1 -> Logical Operator1/2
  MATLAB Function/1(validAppend) -> No HDL/1(In2), Logical Operator2/1, Logical Operator/2
  Data Field Generator/3(frameStartOut) -> Delay2/1
  Data Field Generator/1(pktBits) -> Delay/1
  Data Field Generator/2(pktValid) -> Delay1/1
  BB Header Generator/1(DFLOut) -> Delay4/1
  BB Header Generator/5(endOut) -> Delay8/1
  frameEnd/1 -> Data Field Generator/5(frameEnd)
  SYNC/1 -> BB Header Generator/5(SYNC)
  frameStart/1 -> BB Header Generator/1(startIn), Data Field Generator/6(frameStart)
  BB Header Generator/3(startOut) -> Delay6/1
  dataIn/1 -> Data Field Generator/1(dataIn)
  startIn/1 -> Data Field Generator/2(startIn)
  Data Field Generator/4(frameEndOut) -> Delay3/1
  endIn/1 -> Data Field Generator/3(endIn)
  UPL/1 -> BB Header Generator/4(UPL), Data Field Generator/7(UPL)
  BB Header Generator/4(validOut) -> Delay7/1
  validIn/1 -> No HDL/3(vld), Data Field Generator/4(validIn)
  DFL/1 -> BB Header Generator/3(DFL)
  BB Header Generator/2(bitsOut) -> Delay5/1
  TSorGS/1 -> BB Header Generator/2(TSorGS)
  MATLAB Function/2(endAppend) -> No HDL/2(u)

== system dvbs2hdlTransmitterCore/DVB-S2 Tx/BB Frame Generator/BB Scrambler ==
  bitsIn : Inport
  startIn : Inport  Port=2
  endIn : Inport  Port=3
  validIn : Inport  Port=4
  MODCOD : Inport  Port=5
  FECFrame : Inport  Port=6
  Data Type Conversion : DataTypeConversion  OutDataTypeStr=boolean  SaturateOnIntegerOverflow=off  RndMeth=Floor
  Delay{1..6} (6 alike) : Delay  DelayLength=1
  Logical Operator : Logic  Operator=XOR  AllPortsSameDT=off  OutDataTypeStr=boolean
  Subsystem : Subsystem
  bitsOut : Outport
  startOut : Outport  Port=2
  endOut : Outport  Port=3
  validOut : Outport  Port=4
  MODCODOut : Outport  Port=5
  FECFrameOut : Outport  Port=6
  wires:
  FECFrame/1 -> Delay6/1
  Delay6/1 -> FECFrameOut/1
  Delay4/1 -> MODCODOut/1
  Delay1/1 -> endOut/1
  Delay2/1 -> bitsOut/1
  Delay3/1 -> startOut/1
  Delay5/1 -> validOut/1
  MODCOD/1 -> Delay4/1
  Data Type Conversion/1 -> Logical Operator/1
  Logical Operator/1 -> Delay2/1
  startIn/1 -> Subsystem/1(In1), Delay3/1
  Subsystem/1(Out1) -> Data Type Conversion/1
  validIn/1 -> Subsystem/Enable, Delay5/1
  bitsIn/1 -> Logical Operator/2
  endIn/1 -> Delay1/1

== system dvbs2hdlTransmitterCore/DVB-S2 Tx/BB Frame Generator/Data Store FIFO ==
  pktBits : Inport
  pktValid : Inport  Port=2
  DFLOut : Inport  Port=3
  bitsOut : Inport  Port=4
  startOut : Inport  Port=5
  endOut : Inport  Port=6
  validOut : Inport  Port=7
  MODCOD : Inport  Port=8
  FECFrame : Inport  Port=9
  Delay{,1..14} (15 alike) : Delay  DelayLength=1
  HDL Counter : hdlsllib/Sources/HDL Counter  CountType=Count limited  CountInit=0  CountStep=1  CountMax=2^7-1  CountFromType=Initial value  CountFrom=0  CountResetPort=off  CountLoadPort=off  CountEnbPort=on  CountDirPort=off  CountHitOutputPort=off  CountDataType=Unsigned  CountWordLen=7  CountFracLen=0  CountSampTime=1
  HDL Counter1 : hdlsllib/Sources/HDL Counter  CountType=Count limited  CountInit=0  CountStep=1  CountMax=2^7-1  CountFromType=Initial value  CountFrom=0  CountResetPort=off  CountLoadPort=off  CountEnbPort=on  CountDirPort=off  CountHitOutputPort=off  CountDataType=Unsigned  CountWordLen=7  CountFracLen=0  CountSampTime=1
  MATLAB Function : MATLAB Function  TreatAsAtomicUnit=on
  No HDL : Subsystem
  Simple Dual Port RAM : hdlsllib/HDL RAMs/Simple Dual Port RAM  ram_size=nextpow2(80)
  dataBits : Outport
  dataValid : Outport  Port=2
  dataEnd : Outport  Port=3
  headerBits : Outport  Port=4
  headerStart : Outport  Port=5
  headerValid : Outport  Port=6
  MODCODOut : Outport  Port=7
  FECFrameOut : Outport  Port=8
  wires:
  MATLAB Function/1(validOut) -> No HDL/1(rd), HDL Counter1/1, Delay/1
  Delay13/1 -> Delay14/1
  Delay14/1 -> FECFrameOut/1
  FECFrame/1 -> Delay13/1
  Delay12/1 -> MODCODOut/1
  Delay11/1 -> headerValid/1
  Delay10/1 -> headerStart/1
  Delay9/1 -> headerBits/1
  Delay8/1 -> dataEnd/1
  Delay7/1 -> dataValid/1
  Delay6/1 -> dataBits/1
  Delay5/1 -> Delay12/1
  MODCOD/1 -> Delay5/1
  Delay3/1 -> Delay10/1
  HDL Counter/1 -> Simple Dual Port RAM/2
  Delay4/1 -> Delay11/1
  Delay2/1 -> Delay9/1
  Delay1/1 -> Delay8/1
  Delay/1 -> Delay7/1
  MATLAB Function/2(endOut) -> Delay1/1
  HDL Counter1/1 -> Simple Dual Port RAM/4
  DFLOut/1 -> MATLAB Function/3(DFL)
  validOut/1 -> Delay4/1
  startOut/1 -> Delay3/1
  bitsOut/1 -> Delay2/1
  Simple Dual Port RAM/1 -> Delay6/1
  pktValid/1 -> No HDL/2(wr), HDL Counter/1, Simple Dual Port RAM/3, MATLAB Function/1(wr)
  pktBits/1 -> Simple Dual Port RAM/1
  endOut/1 -> MATLAB Function/2(startIn)

== system dvbs2hdlTransmitterCore/DVB-S2 Tx/BB Frame Generator/Multiplexer ==
  dataBits : Inport
  dataValid : Inport  Port=2
  dataEnd : Inport  Port=3
  headerBits : Inport  Port=4
  headerStart : Inport  Port=5
  headerValid : Inport  Port=6
  MODCOD : Inport  Port=7
  FECFrame : Inport  Port=8
  Delay{,1..3} (4 alike) : Delay
  Delay4 : Delay  DelayLength=1
  Delay5 : Delay  DelayLength=1
  Logical Operator : Logic  Operator=OR  AllPortsSameDT=off  OutDataTypeStr=boolean
  No HDL : Subsystem
  Switch : Switch  Criteria=u2 ~= 0  SaturateOnIntegerOverflow=off  InputSameDT=off
  dataOut : Outport
  startOut : Outport  Port=2
  endOut : Outport  Port=3
  validOut : Outport  Port=4
  MODCODOut : Outport  Port=5
  FECFrameOut : Outport  Port=6
  wires:
  FECFrame/1 -> Delay5/1
  Delay5/1 -> FECFrameOut/1
  Delay4/1 -> MODCODOut/1
  Delay3/1 -> endOut/1
  Delay2/1 -> startOut/1
  Delay1/1 -> validOut/1
  Delay/1 -> dataOut/1
  dataValid/1 -> No HDL/1(dvalid), Logical Operator/1, Switch/2
  MODCOD/1 -> Delay4/1
  Logical Operator/1 -> Delay1/1
  Switch/1 -> Delay/1
  headerValid/1 -> No HDL/2(hvalid), Logical Operator/2
  headerBits/1 -> Switch/3
  dataBits/1 -> Switch/1
  dataEnd/1 -> Delay3/1
  headerStart/1 -> Delay2/1

== system dvbs2hdlTransmitterCore/DVB-S2 Tx/FEC Encoder/DVB-S2 BCH Encoder ==
  dataIn : Inport
  ctrlIn : Inport  Port=2
  frameType : Inport  Port=3
  codeRateIdx : Inport  Port=4
  Input controller : Subsystem
  Output Controller : Subsystem
  Parity Generation : Subsystem
  Store and Retreive Input : Subsystem
  Terminator : Terminator
  dataOut : Outport
  ctrlOut : Outport  Port=2
  wires:
  Store and Retreive Input/2(outrd_data) -> Parity Generation/1(outrd_data)
  Store and Retreive Input/3(outRd_valid) -> Parity Generation/2(outRd_valid)
  Output Controller/1(outData) -> dataOut/1
  Output Controller/2(outCtrl) -> ctrlOut/1
  Store and Retreive Input/4(ParityCalCompFlag) -> Parity Generation/3(ParityCalCompFlag)
  Parity Generation/3(parityScalarOut) -> Output Controller/4(outputParity)
  Parity Generation/4(parityScalarValidOut) -> Output Controller/5(validParity)
  Output Controller/3(nxtFrame) -> Terminator/1
  Input controller/6(reset) -> Store and Retreive Input/7(resetIn)
  ctrlIn/1 -> Input controller/1(ctrlIn)
  frameType/1 -> Input controller/2(frameType)
  codeRateIdx/1 -> Input controller/3(codeRateIdx)
  Input controller/1(iwr_enb) -> Store and Retreive Input/2(iwr_enb)
  Input controller/8(sampledStartIn) -> Output Controller/8(sampledStartIn)
  Input controller/2(iwr_addr) -> Store and Retreive Input/3(iwr_addr)
  Input controller/5(framLenDelayed) -> Store and Retreive Input/6(framLenDelayed)
  Input controller/3(ird_addr) -> Store and Retreive Input/4(ird_addr)
  Input controller/7(parLen) -> Output Controller/7(parLen), Parity Generation/5(parLen)
  Input controller/4(ird_valid) -> Store and Retreive Input/5(ird_valid)
  Input controller/11(frameLen) -> Output Controller/11(frameLen)
  Input controller/12(validCodeRate) -> Output Controller/12(validCodeRate)
  Input controller/13(unitFrameLen) -> Output Controller/13(unitFrameLen)
  dataIn/1 -> Store and Retreive Input/1(iwr_data)
  Store and Retreive Input/5(resetOut) -> Parity Generation/4(resetIn)
  Parity Generation/5(resetOut) -> Output Controller/6(resetIn)
  Parity Generation/1(readDataOut) -> Output Controller/2(outputMsg)
  Parity Generation/2(readValidOut) -> Output Controller/3(validMsg)
  Store and Retreive Input/1(framLenDelay) -> Output Controller/1(framLenDelayed)
  Input controller/9(enbBCHEnc) -> Output Controller/9(enbBCHEnc)
  Input controller/10(sampledEndIn) -> Output Controller/10(sampledEndIn)

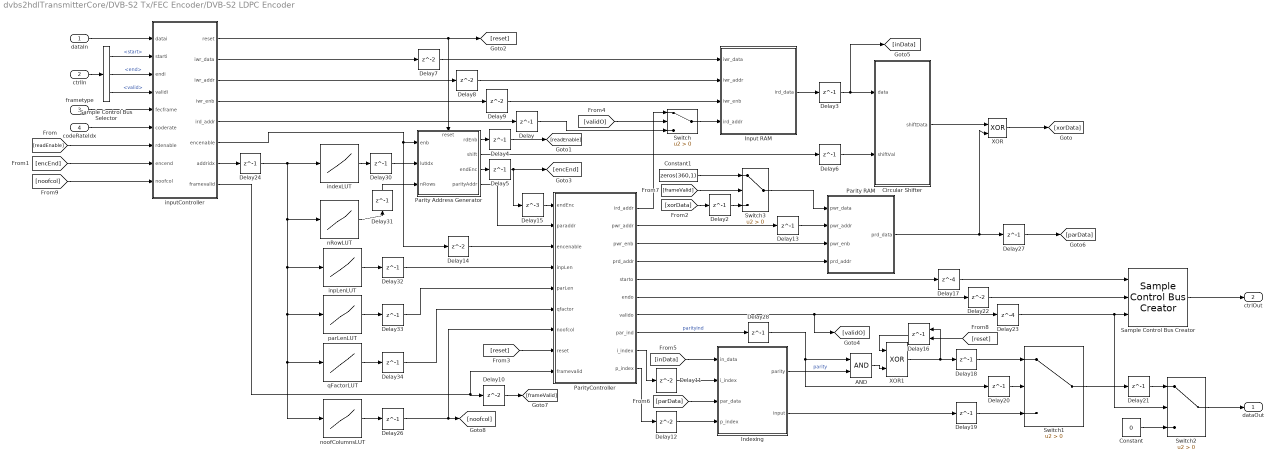
== system dvbs2hdlTransmitterCore/DVB-S2 Tx/FEC Encoder/DVB-S2 LDPC Encoder ==
  dataIn : Inport
  ctrlIn : Inport  Port=2
  frametype : Inport  Port=3
  codeRateIdx : Inport  Port=4
  AND : Logic  IconShape=distinctive  AllPortsSameDT=off  OutDataTypeStr=boolean
  Circular Shifter : Subsystem
  Constant : Constant  Value=0  OutDataTypeStr=boolean  SampleTime=-1
  Constant1 : Constant  Value=zeros(360,1)  OutDataTypeStr=boolean  SampleTime=-1
  Delay{,2..6,13,18..21,24,26..28,30..34} (20 alike) : Delay  DelayLength=1
  Delay{7..10,14,22} (6 alike) : Delay
  Delay11 : Delay  InitialCondition=1
  Delay12 : Delay  InitialCondition=1
  Delay15 : Delay  DelayLength=3
  Delay16 : Delay  DelayLength=1  ExternalReset=Level
      settings: InputPortMap=u0,r5
  Delay17 : Delay  DelayLength=4
  Delay23 : Delay  DelayLength=4  InitialCondition=0
  Indexing : MATLAB Function  TreatAsAtomicUnit=on
  Input RAM : Subsystem  TreatAsAtomicUnit=on
  Parity Address Generator : Subsystem
      settings: PortSchema="{\"entries\":[{\"content\":{\"sides\":[{\"content\":{\"connectorIds\":[\"In1\",\"In2\",\"In3\"]},\"type\":\"ConnectorPlacement.EquallySpacedRectSide\",\"uuid\":\"3d7dec72-7252-434a-9e41-e0042beb8f81\"},{\"content\":{\"connectorIds\":[\"Out1\",\"Out2\",\"Out3\",\"Out4\"],\"side\":\"RIGHT\"},\"type\":\"ConnectorPlacement.EquallySpacedRectSide\",\"uuid\":\"b52d290b-db9d-4f8b-b785-ddc131f6f7c7\"},{\"content\":{\"connectorIds\":[\"In4\"],\"side\":\"TOP\"},\"type\":\"ConnectorPlacement.EquallySpacedRectSide\",\"uuid\":\"6c6734b1-a517-4502-8814-67d54e3edf46\"}]},\"type\":\"ConnectorPlacement.EquallySpacedConnector\",\"uuid\":\"7bd65a32-b8b8-4f3b-b937-2885ab80089c\"}],\"packageUris\":[\"http://schema.mathworks.com/mf0/Connector/R2020b\"],\"version\":\"1.0\"}"
  Parity RAM : Subsystem  TreatAsAtomicUnit=on
  ParityController : MATLAB Function  TreatAsAtomicUnit=on
  Sample Control Bus Creator : whdlutilities/Sample Control Bus Creator
  Sample Control Bus Selector : whdlutilities/Sample Control Bus Selector  OutputSignals=start,end,valid
  Switch{,1..3} (4 alike) : Switch  Criteria=u2 > Threshold  SaturateOnIntegerOverflow=off  InputSameDT=off
  XOR : Logic  Operator=XOR  IconShape=distinctive  AllPortsSameDT=off  OutDataTypeStr=boolean
  XOR1 : Logic  Operator=XOR  IconShape=distinctive  AllPortsSameDT=off  OutDataTypeStr=fixdt(0,1,0)
  indexLUT : Lookup_n-D  NumberOfTableDimensions=1  BreakpointsSpecification=Even spacing  BreakpointsForDimension1=[1:20]  BreakpointsForDimension1FirstPoint=0  Table=[0,45,105,177,267,375,495,630,774,924,1084,1246,1246,1246,1246,1246,1246,1255,1270,1288,1308,1335,1365,1398,1433,1470,1510,1510,1510,1510,1510,1510]  InterpMethod=Flat  RemoveProtectionInput=on  InternalRulePriority=Speed  OutDataTypeStr=fixdt(0,11,0)  RndMeth=Simplest
  inpLenLUT : Lookup_n-D  NumberOfTableDimensions=1  BreakpointsSpecification=Even spacing  BreakpointsForDimension1=[1:20]  BreakpointsForDimension1FirstPoint=0  Table=[16200,21600,25920,32400,38880,43200,48600,51840,54000,57600,58320,58320,58320,58320,58320,58320,3240,5400,6480,7200,9720,10800,11880,12600,13320,14400,14400,14400,14400,14400,14400,14400]  InterpMethod=Flat  RemoveProtectionInput=on  InternalRulePriority=Speed  OutDataTypeStr=fixdt(0,16,0)  RndMeth=Simplest
  inputController : MATLAB Function  TreatAsAtomicUnit=on
  nRowLUT : Lookup_n-D  NumberOfTableDimensions=1  BreakpointsSpecification=Even spacing  BreakpointsForDimension1=[1:20]  BreakpointsForDimension1FirstPoint=0  Table=[45,60,72,90,108,120,135,144,150,160,162,162,162,162,162,162,9,15,18,20,27,30,33,35,37,40,40,40,40,40,40,40]  InterpMethod=Flat  RemoveProtectionInput=on  InternalRulePriority=Speed  OutDataTypeStr=fixdt(0,8,0)  RndMeth=Simplest
  noofColumnsLUT : Lookup_n-D  NumberOfTableDimensions=1  BreakpointsSpecification=Even spacing  BreakpointsForDimension1=[1:20]  BreakpointsForDimension1FirstPoint=0  Table=[45,60,72,90,108,120,135,144,150,160,162,162,162,162,162,162,9,15,18,20,27,30,33,35,37,40,40,40,40,40,40,40]  InterpMethod=Flat  RemoveProtectionInput=on  InternalRulePriority=Speed  OutDataTypeStr=uint8  RndMeth=Simplest
  parLenLUT : Lookup_n-D  NumberOfTableDimensions=1  BreakpointsSpecification=Even spacing  BreakpointsForDimension1=[1:20]  BreakpointsForDimension1FirstPoint=0  Table=[48600,43200,38880,32400,25920,21600,16200,12960,10800,7200,6480,6480,6480,6480,6480,6480,12960,10800,9720,9000,6480,5400,4320,3600,2880,1800,1800,1800,1800,1800,1800,1800]  InterpMethod=Flat  RemoveProtectionInput=on  InternalRulePriority=Speed  OutDataTypeStr=fixdt(0,16,0)  RndMeth=Simplest
  qFactorLUT : Lookup_n-D  NumberOfTableDimensions=1  BreakpointsSpecification=Even spacing  BreakpointsForDimension1=[1:20]  BreakpointsForDimension1FirstPoint=0  Table=[135,120,108,90,72,60,45,36,30,20,18,18,18,18,18,18,36,30,27,25,18,15,12,10,8,5,5,5,5,5,5,5]  InterpMethod=Flat  RemoveProtectionInput=on  InternalRulePriority=Speed  OutDataTypeStr=fixdt(0,9,0)  RndMeth=Simplest
  dataOut : Outport
  ctrlOut : Outport  Port=2
  wires:
  inputController/7(addridx) -> Delay24/1
  codeRateIdx/1 -> inputController/6(coderate)
  ParityController/9(i_index) -> Delay11/1
  Indexing/2(input) -> Delay19/1
  [reset] -> ParityController/8(reset)
  inputController/5(ird_addr) -> Delay/1
  ParityController/6(endo) -> Delay22/1
  Sample Control Bus Selector/1 -> inputController/2(starti)  "<start>"
  Parity Address Generator/3(endEnc) -> Delay5/1
  XOR1/1 -> Delay18/1, Delay16/1
  inputController/4(iwr_enb) -> Delay9/1
  qFactorLUT/1 -> Delay34/1
  Delay18/1 -> Switch1/1
  [reset] -> Delay16/2
  inputController/1(reset) -> [reset], Parity Address Generator/4(reset)
  [parData] -> Indexing/3(par_data)
  Parity Address Generator/1(rdEnb) -> Delay4/1
  inputController/6(encenable) -> Parity Address Generator/1(enb), Delay14/1
  Delay20/1 -> Switch1/2
  ParityController/3(pwr_enb) -> Parity RAM/3(pwr_enb)
  Delay2/1 -> Switch3/3
  Delay7/1 -> Input RAM/1(iwr_data)
  Delay15/1 -> ParityController/1(endEnc)
  Parity Address Generator/2(shift) -> Delay6/1
  Delay12/1 -> Indexing/4(p_index)
  Delay19/1 -> Switch1/3
  Delay4/1 -> [readEnable]
  inputController/2(iwr_data) -> Delay7/1
  Delay21/1 -> Switch2/1
  Delay/1 -> Switch/3
  Constant/1 -> Switch2/3
  nRowLUT/1 -> Delay31/1
  Switch1/1 -> Delay21/1
  ctrlIn/1 -> Sample Control Bus Selector/1
  [encEnd] -> inputController/8(encend)
  [frameValid] -> Switch3/2
  Constant1/1 -> Switch3/1
  [readEnable] -> inputController/7(rdenable)
  AND/1 -> XOR1/2
  dataIn/1 -> inputController/1(datai)
  ParityController/8(par_ind) -> Delay28/1  "parityInd"
  Delay24/1 -> indexLUT/1, nRowLUT/1, inpLenLUT/1, parLenLUT/1, qFactorLUT/1, noofColumnsLUT/1
  inputController/3(iwr_addr) -> Delay8/1
  Delay14/1 -> ParityController/3(encenable)
  Delay16/1 -> XOR1/1
  Switch/1 -> Input RAM/4(ird_addr)
  ParityController/2(pwr_addr) -> Delay13/1
  inpLenLUT/1 -> Delay32/1
  Delay5/1 -> Delay15/1, [encEnd]
  Delay23/1 -> Switch2/2, Sample Control Bus Creator/3
  Delay11/1 -> Indexing/2(i_index)
  Delay31/1 -> Parity Address Generator/3(nRows)
  [inData] -> Indexing/1(in_data)
  ParityController/5(starto) -> Delay17/1
  Delay26/1 -> [noofcol], ParityController/7(noofcol)
  Delay32/1 -> ParityController/4(inpLen)
  ParityController/4(prd_addr) -> Parity RAM/4(prd_addr)
  noofColumnsLUT/1 -> Delay26/1
  inputController/8(framevalid) -> ParityController/9(framevalid), Delay10/1
  Delay34/1 -> ParityController/6(qfactor)
  Switch3/1 -> Parity RAM/1(pwr_data)
  parLenLUT/1 -> Delay33/1
  Delay30/1 -> Parity Address Generator/2(lutIdx)
  XOR/1 -> [xorData]
  indexLUT/1 -> Delay30/1
  frametype/1 -> inputController/5(fecframe)
  Switch2/1 -> dataOut/1
  Parity RAM/1(prd_data) -> XOR/2, Delay27/1
  Delay13/1 -> Parity RAM/2(pwr_addr)
  Indexing/1(parity) -> AND/2  "parity"
  Delay9/1 -> Input RAM/3(iwr_enb)
  Delay17/1 -> Sample Control Bus Creator/1
  [noofcol] -> inputController/9(noofcol)
  [xorData] -> Delay2/1
  Delay33/1 -> ParityController/5(parLen)
  Delay22/1 -> Sample Control Bus Creator/2
  Sample Control Bus Creator/1 -> ctrlOut/1
  [validO] -> Switch/2
  Delay10/1 -> [frameValid]
  ParityController/7(valido) -> Delay23/1, [validO]
  Parity Address Generator/4(parityAddr) -> ParityController/2(paraddr)
  Sample Control Bus Selector/2 -> inputController/3(endi)  "<end>"
  Delay28/1 -> AND/1, Delay20/1
  ParityController/1(ird_addr) -> Switch/1
  Sample Control Bus Selector/3 -> inputController/4(validi)  "<valid>"
  Delay27/1 -> [parData]
  Circular Shifter/1(shiftData) -> XOR/1
  Delay3/1 -> Circular Shifter/1(data), [inData]
  Delay6/1 -> Circular Shifter/2(shiftVal)
  ParityController/10(p_index) -> Delay12/1
  Delay8/1 -> Input RAM/2(iwr_addr)
  Input RAM/1(ird_data) -> Delay3/1
